simulink model "solarPV_grid_04_04"  (R2021a)
settings: Solver=FixedStepAuto  StartTime=0.0  StopTime=5  FixedStep=1e-6  RelTol=1e-3
libraries: spsIGBTDiodeLib x6, spsSeriesRLCBranchLib x6, slpidlib x4, spsCurrentMeasurementLib x4, spsVoltageMeasurementLib x2, simulink x2, spsGroundLib x1, spsPVArrayLib x1, spsdq0toabcLib x1, spsThreePhaseProgrammableVoltageSourceLib x1, spsThreePhaseVIMeasurementLib x1, spspowerguiLib x1
settings Model: Creator=user  LastModifiedBy=Arun Rahul S
settings SolverCC: AlgebraicLoopSolver=TrustRegion
settings DataIOCC: ReturnWorkspaceOutputs=off
settings DebuggingCC: SFMachineParentedDataDiag=warning  ArithmeticOperatorsInVariantConditions=warning
settings SFSimCC: SimUseLocalCustomCode=off  CustomCodeUndefinedFunction=UseInterfaceOnly
settings RTWCC: RTWUseLocalCustomCode=off

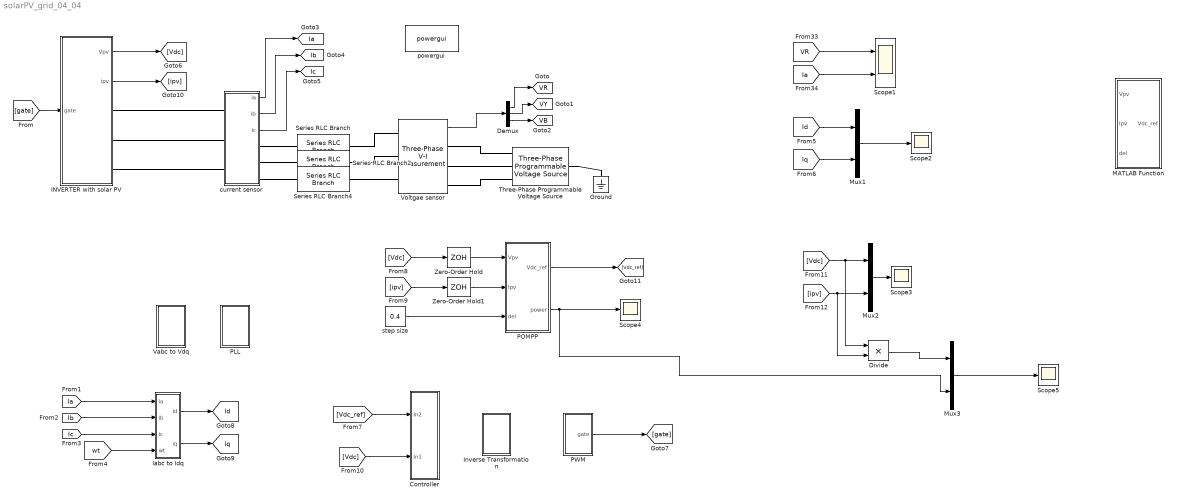
== system solarPV_grid_04_04 ==
  Controller : Subsystem
  Demux : Demux  Outputs=3
  Divide : Product  Inputs=**
  Ground : spsGroundLib/Ground  LConnTagsString=a
  INVERTER with solar PV : Subsystem
  Iabc to Idq : Subsystem
  Inverse Transformation : Subsystem
  MATLAB Function : MATLAB Function  TreatAsAtomicUnit=on
  Mux1 : Mux  Inputs=2
  Mux2 : Mux  Inputs=2
  Mux3 : Mux  Inputs=2
  PLL : Subsystem
  POMPP : MATLAB Function  TreatAsAtomicUnit=on
  PWM : Subsystem
  Scope1 : Scope  NumInputPorts=2
  Scope{2..5} (4 alike) : Scope
  Series RLC Branch : spsSeriesRLCBranchLib/Series RLC Branch  LConnTagsString=__new0  RConnTagsString=__new0  BranchType=RL  Resistance=0.6  Inductance=10e-3  SetiL0=off  InitialCurrent=0  Capacitance=1e-6  Setx0=off  InitialVoltage=0  Measurements=None
  Series RLC Branch2 : spsSeriesRLCBranchLib/Series RLC Branch  LConnTagsString=__new0  RConnTagsString=__new0  BranchType=RL  Resistance=0.6  Inductance=10e-3  SetiL0=off  InitialCurrent=0  Capacitance=1e-6  Setx0=off  InitialVoltage=0  Measurements=None
  Series RLC Branch4 : spsSeriesRLCBranchLib/Series RLC Branch  LConnTagsString=__new0  RConnTagsString=__new0  BranchType=RL  Resistance=0.6  Inductance=10e-3  SetiL0=off  InitialCurrent=0  Capacitance=1e-6  Setx0=off  InitialVoltage=0  Measurements=None
  Three-Phase Programmable Voltage Source : spsThreePhaseProgrammableVoltageSourceLib/Three-Phase Programmable Voltage Source  PositiveSequence="[400  0 50]"  VariationEntity=None  VariationType=Table of time-amplitude pairs  VariationTypeAlt=Step  VariationStep=0.5  VariationRate=10  VariationMagnitude=0.3  VariationFrequency=2  VariationTiming=[1 2]  VariationPhaseA=off  Amplitudes=[1 0.8 1.2 1.0]  TimeValues=[0 0.1 0.15 0.2]  HarmonicGeneration=off  HarmonicA=[3 0.2 -25 0]  HarmonicB=[2 0.15 35 2]  Timing="[0.05  3]"  BusType=swing  Pref=0  Qref=0  Qmin=-inf  Qmax=inf
  Vabc to Vdq : Subsystem
  Voltgae sensor : spsThreePhaseVIMeasurementLib/Three-Phase V-I Measurement  VoltageMeasurement=phase-to-ground  SetLabelV=off  LabelV=Vabc  Vpu=off  VpuLL=off  CurrentMeasurement=no  SetLabelI=off  LabelI=Iabc  Ipu=off  Pbase=100e6  Vbase=500e3  OutputType=Complex  PhasorSimulation=off  PSBequivalent=0
  Zero-Order Hold : ZeroOrderHold  SampleTime=10000e-6
  Zero-Order Hold1 : ZeroOrderHold  SampleTime=10000e-6
  current sensor : Subsystem
  powergui : spspowerguiLib/powergui  Priority=1  SimulationMode=Discrete  SampleTime=1e-6  frequency=60  Iterations=50  frequencyindice=50  Pbase=100e6  ErrMax=1e-4  UnitsV=kV  UnitsW=MW  buscounter=0  FunctionMessages=off  echomessages=off  EnableUseOfTLC=off  CurrentSourceSwitches=off  DisableSnubberDevices=off  DisableRonSwitches=off  DisableVfSwitches=off  DisplayEquations=off  AutomaticDiscreteSolvers=off  SolverType=Tustin/Backward Euler (TBE)  Interpol=off  ExternalGateDelay=off  methode=off  Ts=100  x0status=blocks  SPID=on  SwTol=0  HookPort=off  NonlinearTolerance=1e-4  nMaxIteration=100  ContinueOnMaxIteration=off  RestoreLinks=warning  ResistiveCurrentMeasurement=off  Frange=[0:2:500]  Ylog=off  Xlog=on  ShowGrid=off  save=off  variable=ZData  structure=ScopeData1  ZoomFFT=off  StartTime=0.91  cycles=4  DisplayStyle=1  fundamental=50  FreqAxis=off  MaxFrequency=1000  frequencyindicesteady=1  RmsSteady=1  display=off
  step size : Constant  Value=0.4
  tag scope: Ia=global, Ib=global, Ic=global, Id=global, Iq=global, VB=global, VR=global, VY=global
  wires:
  Demux/1 -> [VR]
  Demux/2 -> [VY]
  Demux/3 -> [VB]
  [VR] -> Scope1/1
  [Ia] -> Scope1/2
  current sensor/1(ia) -> [Ia]
  current sensor/2(ib) -> [Ib]
  current sensor/3(ic) -> [Ic]
  PWM/1(gate) -> [gate]
  [gate] -> INVERTER with solar PV/1(gate)
  [Iq] -> Mux1/2
  Mux1/1 -> Scope2/1
  [Id] -> Mux1/1
  [Ia] -> Iabc to Idq/1(ia)
  [Ib] -> Iabc to Idq/2(ib)
  [Ic] -> Iabc to Idq/3(ic)
  [wt] -> Iabc to Idq/4(wt)
  Iabc to Idq/1(id) -> [Id]
  Iabc to Idq/2(iq) -> [Iq]
  Voltgae sensor/1 -> Demux/1
  INVERTER with solar PV/1(Vpv) -> [Vdc]
  INVERTER with solar PV/2(ipv) -> [ipv]
  step size/1 -> POMPP/3(del)
  [Vdc] -> Zero-Order Hold/1
  [ipv] -> Zero-Order Hold1/1
  POMPP/1(Vdc_ref) -> [Vdc_ref]
  Zero-Order Hold/1 -> POMPP/1(Vpv)
  Zero-Order Hold1/1 -> POMPP/2(Ipv)
  [Vdc_ref] -> Controller/1(In2)
  [Vdc] -> Controller/2(In1)
  [Vdc] -> Divide/1, Mux2/1
  [ipv] -> Divide/2, Mux2/2
  Mux2/1 -> Scope3/1
  POMPP/2(power) -> Mux3/2, Scope4/1
  Divide/1 -> Mux3/1
  Mux3/1 -> Scope5/1
  connections:
  current sensor/LConn2 -- INVERTER with solar PV/RConn2
  current sensor/RConn2 -- Series RLC Branch2/LConn1
  current sensor/LConn3 -- INVERTER with solar PV/RConn3
  Series RLC Branch/LConn1 -- current sensor/RConn1
  Series RLC Branch4/LConn1 -- current sensor/RConn3
  Three-Phase Programmable Voltage Source/LConn1 -- Ground/LConn1
  Voltgae sensor/RConn1 -- Three-Phase Programmable Voltage Source/RConn1
  Voltgae sensor/RConn2 -- Three-Phase Programmable Voltage Source/RConn2
  Voltgae sensor/RConn3 -- Three-Phase Programmable Voltage Source/RConn3
  Series RLC Branch/RConn1 -- Voltgae sensor/LConn1
  Series RLC Branch2/RConn1 -- Voltgae sensor/LConn2
  Series RLC Branch4/RConn1 -- Voltgae sensor/LConn3
  INVERTER with solar PV/RConn1 -- current sensor/LConn1

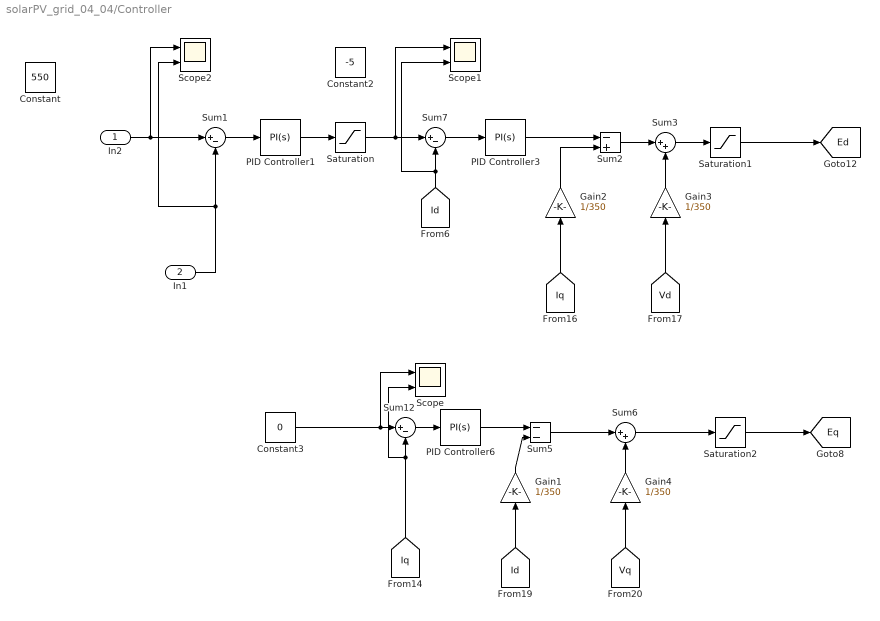
== system solarPV_grid_04_04/Controller ==
  In2 : Inport
  In1 : Inport  Port=2
  Constant : Constant  Value=550
  Constant2 : Constant  Value=-5
  Constant3 : Constant  Value=0
  Gain{1..4} (4 alike) : Gain  Gain=1/350
  PID Controller1 : slpidlib/PID Controller  Controller=PI  Form=Parallel  TimeDomain=Continuous-time  UseExternalTs=off  SampleTime=-1  IntegratorMethod=Forward Euler  FilterMethod=Forward Euler  ControllerParametersSource=internal  P=0.1  I=1  D=0  UseFilter=on  N=100  TunerSelectOption=Transfer Function Based (PID Tuner App)  InitialConditionSource=internal  InitialConditionForIntegrator=0  InitialConditionForFilter=0  DifferentiatorICPrevScaledInput=0  ExternalReset=none  TrackingMode=off  Kt=1  LimitOutput=off  SatLimitsSource=internal  UpperSaturationLimit=inf  LowerSaturationLimit=-inf  LinearizeAsGain=on  AntiWindupMode=none  Kb=1  POutMin=[]  POutMax=[]  IOutMin=[]  IOutMax=[]  DOutMin=[]  DOutMax=[]  NOutMin=[]  NOutMax=[]  SumOutMin=[]  SumOutMax=[]  SaturationOutMin=[]  SaturationOutMax=[]  PParamMin=[]  PParamMax=[]  IParamMin=[]  IParamMax=[]  DParamMin=[]  DParamMax=[]  NParamMin=[]  NParamMax=[]  KbParamMin=[]  KbParamMax=[]  KtParamMin=[]  KtParamMax=[]  KbOutMin=[]  KbOutMax=[]  KtOutMin=[]  KtOutMax=[]  IntegratorOutMin=[]  IntegratorOutMax=[]  FilterOutMin=[]  FilterOutMax=[]  SumI1OutMin=[]  SumI1OutMax=[]  SumI2OutMin=[]  SumI2OutMax=[]  SumI3OutMin=[]  SumI3OutMax=[]  SumI4OutMin=[]  SumI4OutMax=[]  SumDOutMin=[]  SumDOutMax=[]  DifferentiatorOutMin=[]  DifferentiatorOutMax=[]  FilterDiffOutCoefMin=[]  FilterDiffOutCoefMax=[]  ReciprocalOutMin=[]  ReciprocalOutMax=[]  SumDenOutMin=[]  SumDenOutMax=[]  SumNumOutMin=[]  SumNumOutMax=[]  DivideOutMin=[]  DivideOutMax=[]  UdiffTsProdOutMin=[]  UdiffTsProdOutMax=[]  NTsProdOutMin=[]  NTsProdOutMax=[]  UintegralTsProdOutMin=[]  UintegralTsProdOutMax=[]  UngainTsProdOutMin=[]  UngainTsProdOutMax=[]  IntegratorContinuousStateAttributes=''  IntegratorStateMustResolveToSignalObject=off  IntegratorRTWStateStorageClass=Auto  FilterContinuousStateAttributes=''  FilterStateMustResolveToSignalObject=off  FilterRTWStateStorageClass=Auto  ParallelPVariant=InternalParameters  IdealPVariant=Disabled  IVariant=InternalParameters  DVariant=Disabled  IntegratorVariant=Continuous  SatVariant=Disabled  AWVariant=Passthrough  PCopyVariant=Disabled  TRVariant=Disabled  FdbkBlocksVariant=Forward  IdealPFdbkVariant=Disabled  SatFdbkVariant=Disabled  DerivativeFilterVariant=Disabled  NVariant=Disabled  NCopyVariant=Disabled_SignalSpec  FilterICVariant=Disabled  IntegratorICVariant=InternalICs  ExternalResetVariant=Disabled  TRSumVariant=Passthrough  SumFdbkVariant=Disabled  SumVariant=Sum_PI  TsampFilterVariant=InternalTs  TsampNgainVariant=Passthrough  TsampIntegralVariant=Passthrough  ExternalSaturationOutDataTypeStr=Inherit: Same as second input
  PID Controller3 : slpidlib/PID Controller  Controller=PI  Form=Parallel  TimeDomain=Continuous-time  UseExternalTs=off  SampleTime=-1  IntegratorMethod=Forward Euler  FilterMethod=Forward Euler  ControllerParametersSource=internal  P=1  I=1  D=0  UseFilter=on  N=100  TunerSelectOption=Transfer Function Based (PID Tuner App)  InitialConditionSource=internal  InitialConditionForIntegrator=0  InitialConditionForFilter=0  DifferentiatorICPrevScaledInput=0  ExternalReset=none  TrackingMode=off  Kt=1  LimitOutput=off  SatLimitsSource=internal  UpperSaturationLimit=inf  LowerSaturationLimit=-inf  LinearizeAsGain=on  AntiWindupMode=none  Kb=1  POutMin=[]  POutMax=[]  IOutMin=[]  IOutMax=[]  DOutMin=[]  DOutMax=[]  NOutMin=[]  NOutMax=[]  SumOutMin=[]  SumOutMax=[]  SaturationOutMin=[]  SaturationOutMax=[]  PParamMin=[]  PParamMax=[]  IParamMin=[]  IParamMax=[]  DParamMin=[]  DParamMax=[]  NParamMin=[]  NParamMax=[]  KbParamMin=[]  KbParamMax=[]  KtParamMin=[]  KtParamMax=[]  KbOutMin=[]  KbOutMax=[]  KtOutMin=[]  KtOutMax=[]  IntegratorOutMin=[]  IntegratorOutMax=[]  FilterOutMin=[]  FilterOutMax=[]  SumI1OutMin=[]  SumI1OutMax=[]  SumI2OutMin=[]  SumI2OutMax=[]  SumI3OutMin=[]  SumI3OutMax=[]  SumI4OutMin=[]  SumI4OutMax=[]  SumDOutMin=[]  SumDOutMax=[]  DifferentiatorOutMin=[]  DifferentiatorOutMax=[]  FilterDiffOutCoefMin=[]  FilterDiffOutCoefMax=[]  ReciprocalOutMin=[]  ReciprocalOutMax=[]  SumDenOutMin=[]  SumDenOutMax=[]  SumNumOutMin=[]  SumNumOutMax=[]  DivideOutMin=[]  DivideOutMax=[]  UdiffTsProdOutMin=[]  UdiffTsProdOutMax=[]  NTsProdOutMin=[]  NTsProdOutMax=[]  UintegralTsProdOutMin=[]  UintegralTsProdOutMax=[]  UngainTsProdOutMin=[]  UngainTsProdOutMax=[]  IntegratorContinuousStateAttributes=''  IntegratorStateMustResolveToSignalObject=off  IntegratorRTWStateStorageClass=Auto  FilterContinuousStateAttributes=''  FilterStateMustResolveToSignalObject=off  FilterRTWStateStorageClass=Auto  ParallelPVariant=InternalParameters  IdealPVariant=Disabled  IVariant=InternalParameters  DVariant=Disabled  IntegratorVariant=Continuous  SatVariant=Disabled  AWVariant=Passthrough  PCopyVariant=Disabled  TRVariant=Disabled  FdbkBlocksVariant=Forward  IdealPFdbkVariant=Disabled  SatFdbkVariant=Disabled  DerivativeFilterVariant=Disabled  NVariant=Disabled  NCopyVariant=Disabled_SignalSpec  FilterICVariant=Disabled  IntegratorICVariant=InternalICs  ExternalResetVariant=Disabled  TRSumVariant=Passthrough  SumFdbkVariant=Disabled  SumVariant=Sum_PI  TsampFilterVariant=InternalTs  TsampNgainVariant=Passthrough  TsampIntegralVariant=Passthrough  ExternalSaturationOutDataTypeStr=Inherit: Same as second input
  PID Controller6 : slpidlib/PID Controller  Controller=PI  Form=Parallel  TimeDomain=Continuous-time  UseExternalTs=off  SampleTime=-1  IntegratorMethod=Forward Euler  FilterMethod=Forward Euler  ControllerParametersSource=internal  P=1  I=1  D=0  UseFilter=on  N=100  TunerSelectOption=Transfer Function Based (PID Tuner App)  InitialConditionSource=internal  InitialConditionForIntegrator=0  InitialConditionForFilter=0  DifferentiatorICPrevScaledInput=0  ExternalReset=none  TrackingMode=off  Kt=1  LimitOutput=off  SatLimitsSource=internal  UpperSaturationLimit=inf  LowerSaturationLimit=-inf  LinearizeAsGain=on  AntiWindupMode=none  Kb=1  POutMin=[]  POutMax=[]  IOutMin=[]  IOutMax=[]  DOutMin=[]  DOutMax=[]  NOutMin=[]  NOutMax=[]  SumOutMin=[]  SumOutMax=[]  SaturationOutMin=[]  SaturationOutMax=[]  PParamMin=[]  PParamMax=[]  IParamMin=[]  IParamMax=[]  DParamMin=[]  DParamMax=[]  NParamMin=[]  NParamMax=[]  KbParamMin=[]  KbParamMax=[]  KtParamMin=[]  KtParamMax=[]  KbOutMin=[]  KbOutMax=[]  KtOutMin=[]  KtOutMax=[]  IntegratorOutMin=[]  IntegratorOutMax=[]  FilterOutMin=[]  FilterOutMax=[]  SumI1OutMin=[]  SumI1OutMax=[]  SumI2OutMin=[]  SumI2OutMax=[]  SumI3OutMin=[]  SumI3OutMax=[]  SumI4OutMin=[]  SumI4OutMax=[]  SumDOutMin=[]  SumDOutMax=[]  DifferentiatorOutMin=[]  DifferentiatorOutMax=[]  FilterDiffOutCoefMin=[]  FilterDiffOutCoefMax=[]  ReciprocalOutMin=[]  ReciprocalOutMax=[]  SumDenOutMin=[]  SumDenOutMax=[]  SumNumOutMin=[]  SumNumOutMax=[]  DivideOutMin=[]  DivideOutMax=[]  UdiffTsProdOutMin=[]  UdiffTsProdOutMax=[]  NTsProdOutMin=[]  NTsProdOutMax=[]  UintegralTsProdOutMin=[]  UintegralTsProdOutMax=[]  UngainTsProdOutMin=[]  UngainTsProdOutMax=[]  IntegratorContinuousStateAttributes=''  IntegratorStateMustResolveToSignalObject=off  IntegratorRTWStateStorageClass=Auto  FilterContinuousStateAttributes=''  FilterStateMustResolveToSignalObject=off  FilterRTWStateStorageClass=Auto  ParallelPVariant=InternalParameters  IdealPVariant=Disabled  IVariant=InternalParameters  DVariant=Disabled  IntegratorVariant=Continuous  SatVariant=Disabled  AWVariant=Passthrough  PCopyVariant=Disabled  TRVariant=Disabled  FdbkBlocksVariant=Forward  IdealPFdbkVariant=Disabled  SatFdbkVariant=Disabled  DerivativeFilterVariant=Disabled  NVariant=Disabled  NCopyVariant=Disabled_SignalSpec  FilterICVariant=Disabled  IntegratorICVariant=InternalICs  ExternalResetVariant=Disabled  TRSumVariant=Passthrough  SumFdbkVariant=Disabled  SumVariant=Sum_PI  TsampFilterVariant=InternalTs  TsampNgainVariant=Passthrough  TsampIntegralVariant=Passthrough  ExternalSaturationOutDataTypeStr=Inherit: Same as second input
  Saturation : Saturate  UpperLimit=10  LowerLimit=-10
  Saturation1 : Saturate  UpperLimit=1.2  LowerLimit=-1.2
  Saturation2 : Saturate  UpperLimit=1.2  LowerLimit=-1.2
  Scope : Scope  NumInputPorts=2
  Scope1 : Scope  NumInputPorts=2
  Scope2 : Scope  NumInputPorts=2
  Sum1 : Sum  Inputs=|+-
  Sum12 : Sum  Inputs=|+-
  Sum2 : Sum  Inputs=-+
  Sum3 : Sum  Inputs=|++
  Sum5 : Sum  Inputs=--
  Sum6 : Sum  Inputs=|++
  Sum7 : Sum  Inputs=|+-
  tag scope: Ed=global, Eq=global
  wires:
  [Id] -> Scope1/2, Sum7/2
  [Id] -> Gain1/1
  In1/1 -> Scope2/2, Sum1/2
  Sum2/1 -> Sum3/1
  Sum1/1 -> PID Controller1/1
  [Iq] -> Scope/2, Sum12/2
  Sum12/1 -> PID Controller6/1
  Constant3/1 -> Scope/1, Sum12/1
  Sum7/1 -> PID Controller3/1
  Sum6/1 -> Saturation2/1
  Sum5/1 -> Sum6/1
  Sum3/1 -> Saturation1/1
  PID Controller3/1 -> Sum2/1
  PID Controller6/1 -> Sum5/1
  [Iq] -> Gain2/1
  Saturation1/1 -> [Ed]
  Saturation2/1 -> [Eq]
  [Vd] -> Gain3/1
  Gain3/1 -> Sum3/2
  [Vq] -> Gain4/1
  Gain4/1 -> Sum6/2
  Gain2/1 -> Sum2/2
  Gain1/1 -> Sum5/2
  PID Controller1/1 -> Saturation/1
  Saturation/1 -> Scope1/1, Sum7/1
  In2/1 -> Scope2/1, Sum1/1

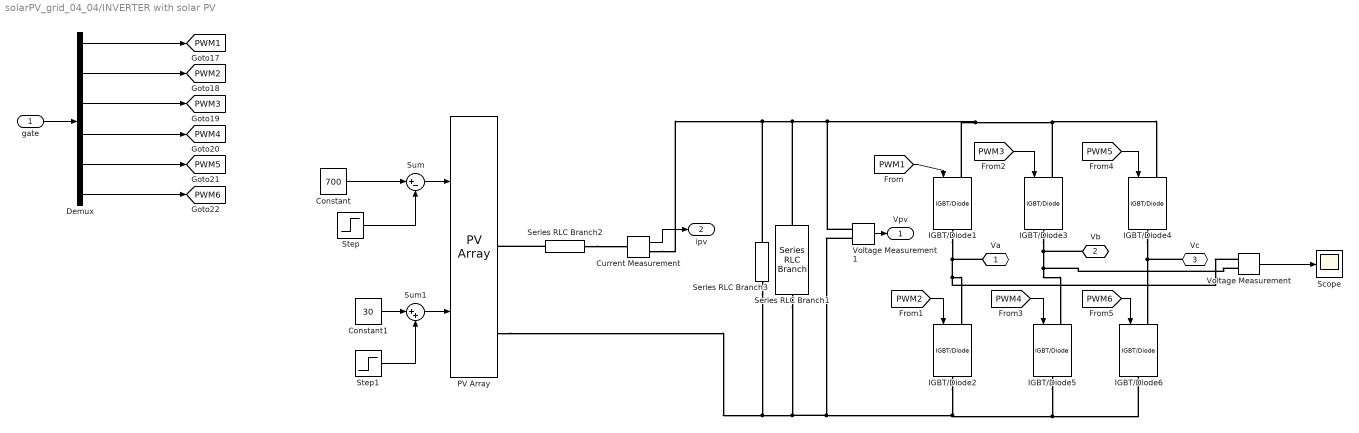
== system solarPV_grid_04_04/INVERTER with solar PV ==
  gate : Inport
  Constant : Constant  Value=700
  Constant1 : Constant  Value=30
  Current Measurement : spsCurrentMeasurementLib/Current Measurement  PhasorSimulation=off  OutputType=Complex  PSBequivalent=0
  Demux : Demux  Outputs=6
  IGBT/Diode{1..6} (6 alike) : spsIGBTDiodeLib/IGBT//Diode  Ron=1e-3  Rs=1e5  Cs=inf  Measurements=off
  PV Array : spsPVArrayLib/PV Array  Npar=1  Nser=24  PlotType=array @ 1000 W/m2 & specified temperatures  S_vec="[ 1000  500  100 ]"  Temp_C_vec="[ 45 25  ]"  ModuleName=User-defined  PlotWhenSelected=off  Pm=213.15  Ncell=60  Voc=36.3  Isc=7.84  Vm=29  Im=7.35  beta_Voc_pc=-0.36099  alpha_Isc_pc=0.102  beta_Voc=-0.13104  alpha_Isc=0.0079968  IL=7.8654  I0=2.9273e-10  nI=0.98119  Rsh=313.0553  Rs=0.39381  RobustModel=off  RobustCellTemperature=313.3991  BAL=on  Tc=1e-6  Tfilter=5e-5
  Scope : Scope
  Series RLC Branch1 : spsSeriesRLCBranchLib/Series RLC Branch  LConnTagsString=__new0  RConnTagsString=__new0  BranchType=RC  Resistance=0.1  Inductance=1e-3  SetiL0=off  InitialCurrent=0  Capacitance=2200e-6  Setx0=on  InitialVoltage=24*36.3  Measurements=Branch voltage
  Series RLC Branch2 : spsSeriesRLCBranchLib/Series RLC Branch  LConnTagsString=__new0  RConnTagsString=__new0  BranchType=R  Resistance=0.5  Inductance=1e-3  SetiL0=off  InitialCurrent=0  Capacitance=4400e-6  Setx0=off  InitialVoltage=0  Measurements=Branch voltage
  Series RLC Branch3 : spsSeriesRLCBranchLib/Series RLC Branch  LConnTagsString=__new0  RConnTagsString=__new0  BranchType=R  Resistance=1000  Inductance=1e-3  SetiL0=off  InitialCurrent=0  Capacitance=4400e-6  Setx0=off  InitialVoltage=0  Measurements=Branch voltage
  Step : Step  Time=3  After=200  SampleTime=0
  Step1 : Step  Time=4  After=10  SampleTime=0
  Sum : Sum  Inputs=|+-
  Sum1 : Sum  Inputs=|++
  Voltage Measurement : spsVoltageMeasurementLib/Voltage Measurement  PhasorSimulation=off  OutputType=Complex  PSBequivalent=0
  Voltage Measurement1 : spsVoltageMeasurementLib/Voltage Measurement  PhasorSimulation=off  OutputType=Complex  PSBequivalent=0
  Va : PMIOPort  Side=Right
  Vb : PMIOPort  Port=2  Side=Right
  Vc : PMIOPort  Port=3  Side=Right
  Vpv : Outport
  ipv : Outport  Port=2
  tag scope: PWM1=global, PWM2=global, PWM3=global, PWM4=global, PWM5=global, PWM6=global
  wires:
  [PWM2] -> IGBT/Diode2/1
  [PWM6] -> IGBT/Diode6/1
  [PWM4] -> IGBT/Diode5/1
  [PWM5] -> IGBT/Diode4/1
  [PWM3] -> IGBT/Diode3/1
  Voltage Measurement/1 -> Scope/1
  gate/1 -> Demux/1
  [PWM1] -> IGBT/Diode1/1
  Demux/1 -> [PWM1]
  Demux/2 -> [PWM2]
  Demux/3 -> [PWM3]
  Demux/4 -> [PWM4]
  Demux/5 -> [PWM5]
  Demux/6 -> [PWM6]
  Current Measurement/1 -> ipv/1
  Sum/1 -> PV Array/1
  Constant/1 -> Sum/1
  Step/1 -> Sum/2
  Constant1/1 -> Sum1/1
  Step1/1 -> Sum1/2
  Sum1/1 -> PV Array/2
  Voltage Measurement1/1 -> Vpv/1
  connections:
  IGBT/Diode3/RConn1 -- Vb/RConn1 -- Voltage Measurement/LConn2 -- IGBT/Diode5/LConn1
  IGBT/Diode2/RConn1 -- Voltage Measurement1/LConn2 -- PV Array/RConn2 -- Series RLC Branch3/RConn1 -- Series RLC Branch1/RConn1 -- IGBT/Diode5/RConn1 -- IGBT/Diode6/RConn1
  IGBT/Diode4/RConn1 -- Vc/RConn1 -- IGBT/Diode6/LConn1
  IGBT/Diode1/RConn1 -- Voltage Measurement/LConn1 -- IGBT/Diode2/LConn1 -- Va/RConn1
  IGBT/Diode3/LConn1 -- Series RLC Branch1/LConn1 -- Series RLC Branch3/LConn1 -- Current Measurement/RConn1 -- Voltage Measurement1/LConn1 -- IGBT/Diode1/LConn1 -- IGBT/Diode4/LConn1
  Series RLC Branch2/RConn1 -- PV Array/RConn1
  Series RLC Branch2/LConn1 -- Current Measurement/LConn1

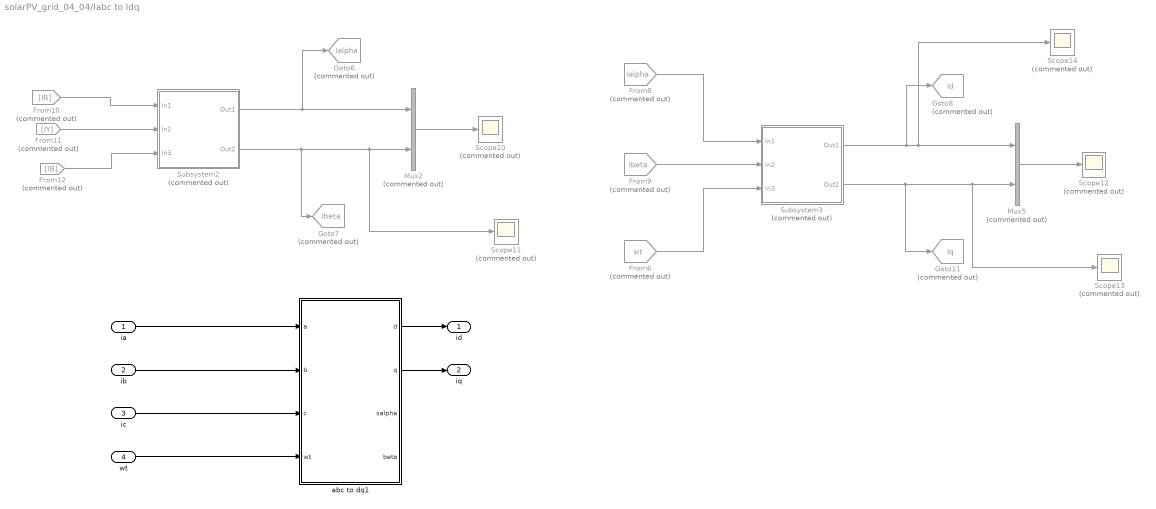
== system solarPV_grid_04_04/Iabc to Idq ==
  ia : Inport
  ib : Inport  Port=2
  ic : Inport  Port=3
  wt : Inport  Port=4
  From10 : From  Commented=on  GotoTag=IR  TagVisibility=global
  From11 : From  Commented=on  GotoTag=IY  TagVisibility=global
  From12 : From  Commented=on  GotoTag=IB  TagVisibility=global
  From6 : From  Commented=on  GotoTag=wt  TagVisibility=global
  From8 : From  Commented=on  GotoTag=Ialpha  TagVisibility=global
  From9 : From  Commented=on  GotoTag=Ibeta  TagVisibility=global
  Goto11 : Goto  Commented=on  GotoTag=Iq  TagVisibility=global
  Goto6 : Goto  Commented=on  GotoTag=Ialpha  TagVisibility=global
  Goto7 : Goto  Commented=on  GotoTag=Ibeta  TagVisibility=global
  Goto8 : Goto  Commented=on  GotoTag=Id  TagVisibility=global
  Mux2 : Mux  Commented=on  Inputs=2
  Mux5 : Mux  Commented=on  Inputs=2
  Scope{10..14} (5 alike) : Scope  Commented=on
  Subsystem2 : Subsystem  Commented=on
  Subsystem3 : Subsystem  Commented=on
  abc to dq1 : Subsystem
  id : Outport
  iq : Outport  Port=2
  wires:
  Subsystem2/2(Out2) -> Goto7/1, Scope11/1, Mux2/2
  From8/1 -> Subsystem3/1(In1)
  From10/1 -> Subsystem2/1(In1)
  Mux5/1 -> Scope12/1
  Subsystem2/1(Out1) -> Goto6/1, Mux2/1
  From11/1 -> Subsystem2/2(In2)
  Subsystem3/1(Out1) -> Goto8/1, Scope14/1, Mux5/1
  From6/1 -> Subsystem3/3(In3)
  Subsystem3/2(Out2) -> Goto11/1, Scope13/1, Mux5/2
  From9/1 -> Subsystem3/2(In2)
  Mux2/1 -> Scope10/1
  From12/1 -> Subsystem2/3(In3)
  ia/1 -> abc to dq1/1(a)
  ib/1 -> abc to dq1/2(b)
  ic/1 -> abc to dq1/3(c)
  wt/1 -> abc to dq1/4(wt)
  abc to dq1/2(q) -> iq/1
  abc to dq1/1(d) -> id/1

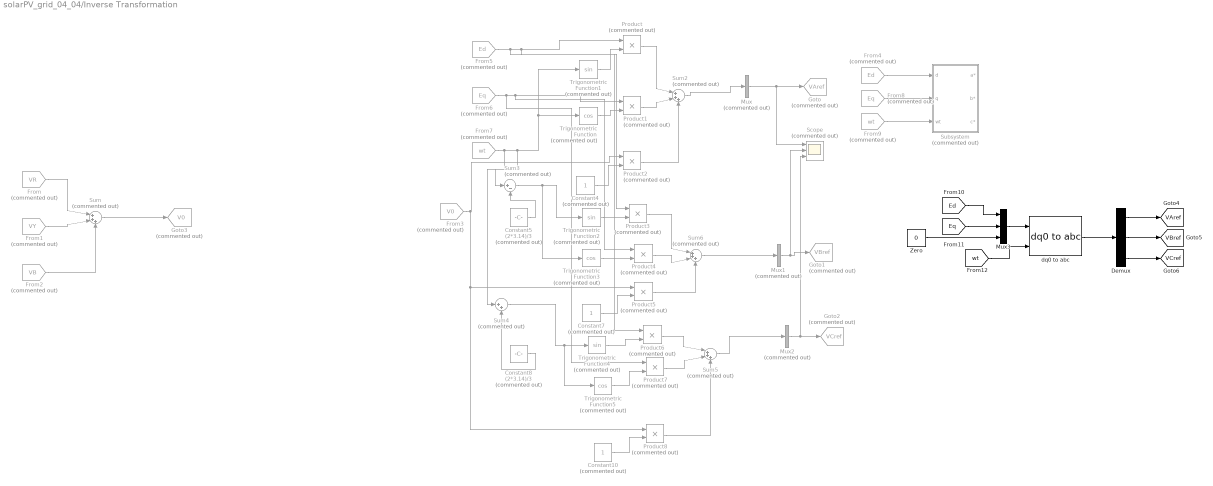
== system solarPV_grid_04_04/Inverse Transformation ==
  Constant10 : Constant  Commented=on
  Constant4 : Constant  Commented=on
  Constant5 : Constant  Commented=on  Value=(2*3.14)/3
  Constant7 : Constant  Commented=on
  Constant8 : Constant  Commented=on  Value=(2*3.14)/3
  Demux : Demux  Outputs=3
  From : From  Commented=on  GotoTag=VR  TagVisibility=global
  From1 : From  Commented=on  GotoTag=VY  TagVisibility=global
  From2 : From  Commented=on  GotoTag=VB  TagVisibility=global
  From3 : From  Commented=on  GotoTag=V0  TagVisibility=global
  From4 : From  Commented=on  GotoTag=Ed  TagVisibility=global
  From5 : From  Commented=on  GotoTag=Ed  TagVisibility=global
  From6 : From  Commented=on  GotoTag=Eq  TagVisibility=global
  From7 : From  Commented=on  GotoTag=wt  TagVisibility=global
  From8 : From  Commented=on  GotoTag=Eq  TagVisibility=global
  From9 : From  Commented=on  GotoTag=wt  TagVisibility=global
  Goto : Goto  Commented=on  GotoTag=VAref  TagVisibility=global
  Goto1 : Goto  Commented=on  GotoTag=VBref  TagVisibility=global
  Goto2 : Goto  Commented=on  GotoTag=VCref  TagVisibility=global
  Goto3 : Goto  Commented=on  GotoTag=V0  TagVisibility=global
  Mux : Mux  Commented=on  Inputs=1
  Mux1 : Mux  Commented=on  Inputs=1
  Mux2 : Mux  Commented=on  Inputs=1
  Mux3 : Mux  Inputs=3
  Product{,1..8} (9 alike) : Product  Commented=on
  Scope : Scope  Commented=on  NumInputPorts=3
  Subsystem : Subsystem  Commented=on
  Sum{,2,5..6} (4 alike) : Sum  Commented=on  Inputs=|+++
  Sum3 : Sum  Commented=on  Inputs=|+-
  Sum4 : Sum  Commented=on  Inputs=|++
  Trigonometric Function : Trigonometry  Commented=on  Operator=cos
  Trigonometric Function1 : Trigonometry  Commented=on
  Trigonometric Function2 : Trigonometry  Commented=on
  Trigonometric Function3 : Trigonometry  Commented=on  Operator=cos
  Trigonometric Function4 : Trigonometry  Commented=on
  Trigonometric Function5 : Trigonometry  Commented=on  Operator=cos
  Zero : Constant  Value=0
  dq0 to abc : spsdq0toabcLib/dq0 to abc  Alignment=Aligned with phase A axis
  tag scope: VAref=global, VBref=global, VCref=global
  wires:
  Constant5/1 -> Sum3/2
  Product5/1 -> Sum6/3
  Trigonometric Function/1 -> Product1/2
  From6/1 -> Product7/1, Product4/1, Product1/1
  From5/1 -> Product6/1, Product3/1, Product/1
  Constant10/1 -> Product8/2
  Constant4/1 -> Product2/2
  Product4/1 -> Sum6/2
  Sum3/1 -> Trigonometric Function3/1, Trigonometric Function2/1
  Trigonometric Function2/1 -> Product3/2
  Product3/1 -> Sum6/1
  Trigonometric Function1/1 -> Product/2
  From7/1 -> Sum3/1, Sum4/1, Trigonometric Function/1, Trigonometric Function1/1
  Trigonometric Function5/1 -> Product7/2
  Product1/1 -> Sum2/2
  Product6/1 -> Sum5/1
  Product2/1 -> Sum2/3
  Product/1 -> Sum2/1
  Trigonometric Function4/1 -> Product6/2
  Constant7/1 -> Product5/2
  Sum4/1 -> Trigonometric Function5/1, Trigonometric Function4/1
  Product7/1 -> Sum5/2
  Trigonometric Function3/1 -> Product4/2
  Constant8/1 -> Sum4/2
  Product8/1 -> Sum5/3
  Sum2/1 -> Mux/1
  Sum6/1 -> Mux1/1
  Sum5/1 -> Mux2/1
  Mux/1 -> Scope/1, Goto/1
  Mux1/1 -> Scope/2, Goto1/1
  Mux2/1 -> Scope/3, Goto2/1
  From/1 -> Sum/1
  From1/1 -> Sum/2
  From2/1 -> Sum/3
  Sum/1 -> Goto3/1
  From3/1 -> Product8/1, Product5/1, Product2/1
  From4/1 -> Subsystem/1(d)
  From8/1 -> Subsystem/2(q)
  From9/1 -> Subsystem/3(wt)
  Mux3/1 -> dq0 to abc/1
  Zero/1 -> Mux3/3
  [wt] -> dq0 to abc/2
  Demux/2 -> [VBref]
  Demux/1 -> [VAref]
  Demux/3 -> [VCref]
  dq0 to abc/1 -> Demux/1
  [Eq] -> Mux3/2
  [Ed] -> Mux3/1

== system solarPV_grid_04_04/PLL ==
  PLL : Subsystem
  tag scope: w=global, wt=global
  wires:
  [Vd] -> ?
  [Vq] -> PLL/1(vq)
  PLL/1(theta) -> [wt]
  PLL/2(w) -> [w]

== system solarPV_grid_04_04/PWM ==
  Mux : Mux  Inputs=6
  SVPWM : Subsystem  Commented=on
  Subsystem : Subsystem
  gate : Outport  VectorParamsAs1DForOutWhenUnconnected=off
  wires:
  [VCref] -> Subsystem/3(VCref)
  [VAref] -> Subsystem/1("VAref ")
  [VBref] -> Subsystem/2(VBref)
  Subsystem/1(PWM1) -> Mux/1
  Subsystem/2(PWM2) -> Mux/2
  Subsystem/3(PWM3) -> Mux/3
  Subsystem/4(PWM4) -> Mux/4
  Subsystem/5(PWM5) -> Mux/5
  Subsystem/6(PWM6) -> Mux/6
  Mux/1 -> gate/1

== system solarPV_grid_04_04/Vabc to Vdq ==
  From10 : From  Commented=on  GotoTag=wt  TagVisibility=global
  From8 : From  Commented=on  GotoTag=Valpha
  From9 : From  Commented=on  GotoTag=Vbeta
  Mux5 : Mux  Inputs=2
  Scope12 : Scope
  Subsystem3 : Subsystem  Commented=on
  abc to dq1 : Subsystem
  tag scope: Vd=global, Vq=global
  wires:
  From9/1 -> Subsystem3/2(In2)
  From8/1 -> Subsystem3/1(In1)
  From10/1 -> Subsystem3/3(In3)
  Mux5/1 -> Scope12/1
  [VR] -> abc to dq1/1(Vsa)
  [VY] -> abc to dq1/2(Vsb)
  [VB] -> abc to dq1/3(Vsc)
  [wt] -> abc to dq1/4(speed(w))
  [Vd] -> Mux5/1
  [Vq] -> Mux5/2
  abc to dq1/2(Vsq) -> [Vq]
  abc to dq1/1(Vsd) -> [Vd]

== system solarPV_grid_04_04/current sensor ==
  Current Measurement : spsCurrentMeasurementLib/Current Measurement  PhasorSimulation=off  OutputType=Complex  PSBequivalent=0
  Current Measurement1 : spsCurrentMeasurementLib/Current Measurement  PhasorSimulation=off  OutputType=Complex  PSBequivalent=0
  Current Measurement2 : spsCurrentMeasurementLib/Current Measurement  PhasorSimulation=off  OutputType=Complex  PSBequivalent=0
  a : PMIOPort  Side=Left
  a' : PMIOPort  Port=2  Side=Right
  b : PMIOPort  Port=3  Side=Left
  b' : PMIOPort  Port=4  Side=Right
  c : PMIOPort  Port=5  Side=Left
  c' : PMIOPort  Port=6  Side=Right
  ia : Outport
  ib : Outport  Port=2
  ic : Outport  Port=3
  wires:
  Current Measurement2/1 -> ic/1
  Current Measurement1/1 -> ib/1
  Current Measurement/1 -> ia/1
  connections:
  Current Measurement/RConn1 -- a/RConn1
  Current Measurement/LConn1 -- a'/RConn1
  b/RConn1 -- Current Measurement1/RConn1
  Current Measurement1/LConn1 -- b'/RConn1
  Current Measurement2/LConn1 -- c'/RConn1
  c/RConn1 -- Current Measurement2/RConn1

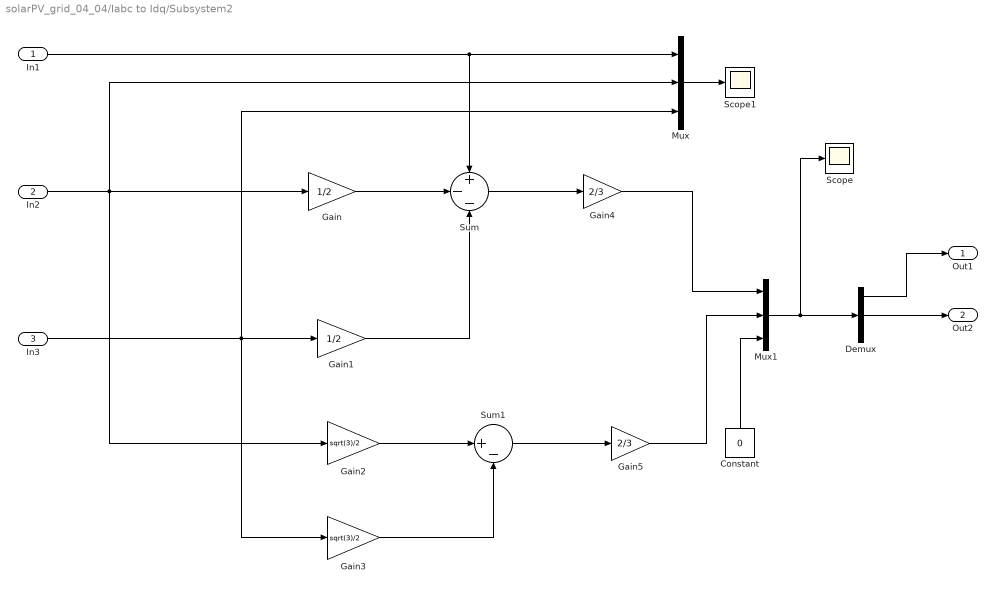
== system solarPV_grid_04_04/Iabc to Idq/Subsystem2 ==
  In1 : Inport
  In2 : Inport  Port=2
  In3 : Inport  Port=3
  Constant : Constant  Value=0
  Demux : Demux  Outputs=3
  Gain : Gain  Gain=1/2
  Gain1 : Gain  Gain=1/2
  Gain2 : Gain  Gain=sqrt(3)/2
  Gain3 : Gain  Gain=sqrt(3)/2
  Gain4 : Gain  Gain=2/3
  Gain5 : Gain  Gain=2/3
  Mux : Mux  Inputs=3
  Mux1 : Mux  Inputs=3
  Scope : Scope
  Scope1 : Scope
  Sum : Sum  Inputs=+--
  Sum1 : Sum  Inputs=|+-
  Out1 : Outport  VectorParamsAs1DForOutWhenUnconnected=off
  Out2 : Outport  Port=2  VectorParamsAs1DForOutWhenUnconnected=off
  wires:
  In1/1 -> Sum/1, Mux/1
  In2/1 -> Gain2/1, Mux/2, Gain/1
  In3/1 -> Mux/3, Gain3/1, Gain1/1
  Gain/1 -> Sum/2
  Sum/1 -> Gain4/1
  Sum1/1 -> Gain5/1
  Gain1/1 -> Sum/3
  Gain2/1 -> Sum1/1
  Gain3/1 -> Sum1/2
  Gain4/1 -> Mux1/1
  Gain5/1 -> Mux1/2
  Constant/1 -> Mux1/3
  Mux1/1 -> Scope/1, Demux/1
  Demux/1 -> Out1/1
  Demux/2 -> Out2/1
  Mux/1 -> Scope1/1

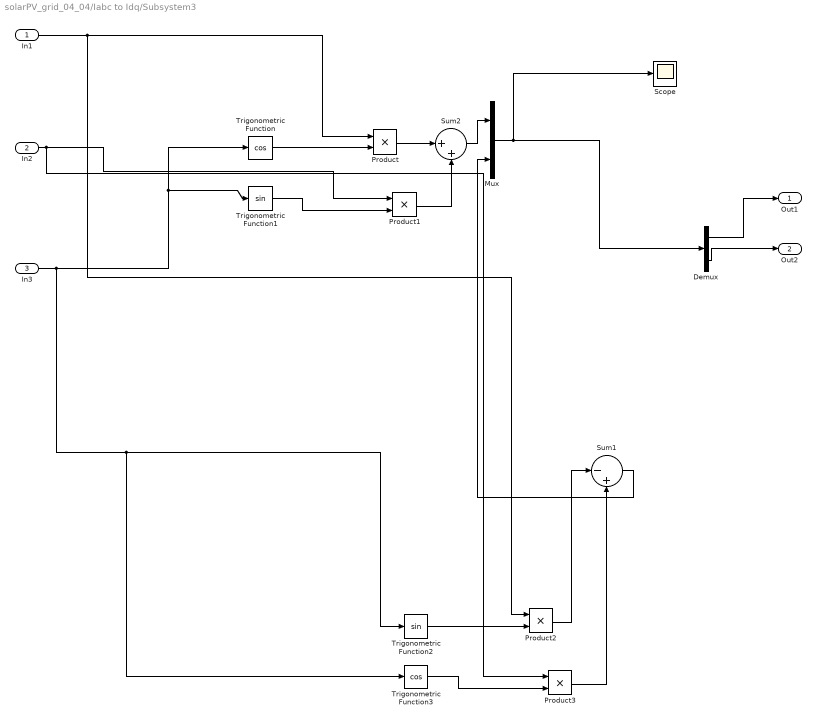
== system solarPV_grid_04_04/Iabc to Idq/Subsystem3 ==
  In1 : Inport
  In2 : Inport  Port=2
  In3 : Inport  Port=3
  Demux : Demux  Outputs=2
  Mux : Mux  Inputs=2
  Product{,1..3} (4 alike) : Product
  Scope : Scope
  Sum1 : Sum  Inputs=|-+
  Sum2 : Sum  Inputs=|++
  Trigonometric Function : Trigonometry  Operator=cos
  Trigonometric Function1 : Trigonometry
  Trigonometric Function2 : Trigonometry
  Trigonometric Function3 : Trigonometry  Operator=cos
  Out1 : Outport  VectorParamsAs1DForOutWhenUnconnected=off
  Out2 : Outport  Port=2  VectorParamsAs1DForOutWhenUnconnected=off
  wires:
  Demux/1 -> Out1/1
  Demux/2 -> Out2/1
  In3/1 -> Trigonometric Function3/1, Trigonometric Function2/1, Trigonometric Function1/1, Trigonometric Function/1
  Trigonometric Function/1 -> Product/2
  Product/1 -> Sum2/1
  In2/1 -> Product3/1, Product1/1
  Trigonometric Function1/1 -> Product1/2
  Product1/1 -> Sum2/2
  Product3/1 -> Sum1/2
  Product2/1 -> Sum1/1
  Trigonometric Function3/1 -> Product3/2
  Trigonometric Function2/1 -> Product2/2
  In1/1 -> Product2/1, Product/1
  Mux/1 -> Scope/1, Demux/1
  Sum2/1 -> Mux/1
  Sum1/1 -> Mux/2

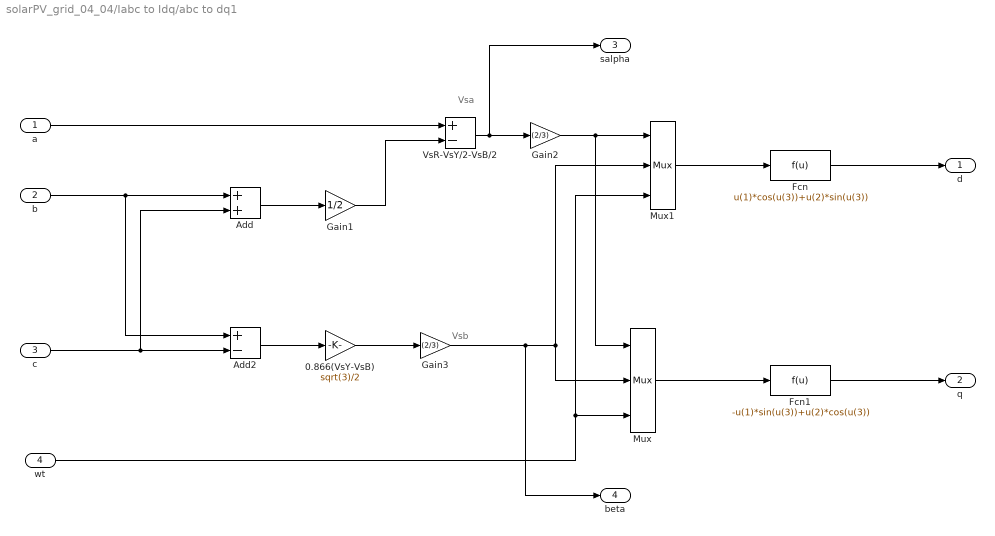
== system solarPV_grid_04_04/Iabc to Idq/abc to dq1 ==
  note: Vsa
  note: Vsb
  a : Inport
  b : Inport  Port=2
  c : Inport  Port=3
  wt : Inport  Port=4
  0.866(VsY-VsB) : Gain  Gain=sqrt(3)/2
  Add : Sum
  Add2 : Sum  Inputs=+-
  Fcn : Fcn  Expr=u(1)*cos(u(3))+u(2)*sin(u(3))
  Fcn1 : Fcn  Expr=-u(1)*sin(u(3))+u(2)*cos(u(3))
  Gain1 : Gain  Gain=1/2
  Gain2 : Gain  Gain=(2/3)
  Gain3 : Gain  Gain=(2/3)
  Mux : Mux  Inputs=3
  Mux1 : Mux  Inputs=3
  VsR-VsY/2-VsB/2 : Sum  Inputs=+-
  d : Outport
  q : Outport  Port=2
  salpha : Outport  Port=3
  beta : Outport  Port=4
  wires:
  wt/1 -> Mux/3, Mux1/3
  VsR-VsY/2-VsB/2/1 -> Gain2/1, salpha/1
  0.866(VsY-VsB)/1 -> Gain3/1
  Fcn1/1 -> q/1
  Fcn/1 -> d/1
  b/1 -> Add/1, Add2/1
  a/1 -> VsR-VsY/2-VsB/2/1
  c/1 -> Add2/2, Add/2
  Add2/1 -> 0.866(VsY-VsB)/1
  Add/1 -> Gain1/1
  Gain1/1 -> VsR-VsY/2-VsB/2/2
  Mux/1 -> Fcn1/1
  Mux1/1 -> Fcn/1
  Gain2/1 -> Mux1/1, Mux/1
  Gain3/1 -> Mux/2, Mux1/2, beta/1

== system solarPV_grid_04_04/Inverse Transformation/Subsystem ==
  d : Inport
  q : Inport  Port=2
  wt : Inport  Port=3
  Fcn : Fcn  Expr=u(1)*cos(u(3))-u(2)*sin(u(3))
  Fcn1 : Fcn  Expr=u(1)*sin(u(3))+u(2)*cos(u(3))
  Fcn2 : Fcn  Expr=u(1)*(2/3)
  Fcn3 : Fcn  Expr=-u(1)*(1/3)+(1/sqrt(3))*u(2)
  Fcn4 : Fcn  Expr=-u(1)*(1/3)-(1/sqrt(3))*u(2)
  Mux : Mux  Inputs=3
  Mux1 : Mux  Inputs=3
  Mux2 : Mux  Inputs=2
  Mux3 : Mux  Inputs=2
  a* : Outport
  b* : Outport  Port=2
  c* : Outport  Port=3
  wires:
  Mux/1 -> Fcn/1
  q/1 -> Mux/2, Mux1/2
  Mux1/1 -> Fcn1/1
  d/1 -> Mux/1, Mux1/1
  wt/1 -> Mux1/3, Mux/3
  Fcn/1 -> Mux2/1, Mux3/1, Fcn2/1
  Mux2/1 -> Fcn3/1
  Fcn1/1 -> Mux3/2, Mux2/2
  Mux3/1 -> Fcn4/1
  Fcn4/1 -> c*/1
  Fcn2/1 -> a*/1
  Fcn3/1 -> b*/1

== system solarPV_grid_04_04/PLL/PLL ==
  vq : Inport
  Constant3 : Constant  Value=2*pi
  Integrator : Integrator
  Mod : Math  Operator=mod  SignedPower=on  SaturateOnIntegerOverflow=on
  PID Controller : slpidlib/PID Controller  Controller=PI  Form=Parallel  TimeDomain=Continuous-time  UseExternalTs=off  SampleTime=-1  IntegratorMethod=Forward Euler  FilterMethod=Forward Euler  ControllerParametersSource=internal  P=10.69499844156994  I=20.78607806516402  D=0  UseFilter=on  N=100  TunerSelectOption=Transfer Function Based (PID Tuner App)  InitialConditionSource=internal  InitialConditionForIntegrator=0  InitialConditionForFilter=0  DifferentiatorICPrevScaledInput=0  ExternalReset=none  TrackingMode=off  Kt=1  LimitOutput=off  SatLimitsSource=internal  UpperSaturationLimit=inf  LowerSaturationLimit=-inf  LinearizeAsGain=on  AntiWindupMode=none  Kb=1  POutMin=[]  POutMax=[]  IOutMin=[]  IOutMax=[]  DOutMin=[]  DOutMax=[]  NOutMin=[]  NOutMax=[]  SumOutMin=[]  SumOutMax=[]  SaturationOutMin=[]  SaturationOutMax=[]  PParamMin=[]  PParamMax=[]  IParamMin=[]  IParamMax=[]  DParamMin=[]  DParamMax=[]  NParamMin=[]  NParamMax=[]  KbParamMin=[]  KbParamMax=[]  KtParamMin=[]  KtParamMax=[]  KbOutMin=[]  KbOutMax=[]  KtOutMin=[]  KtOutMax=[]  IntegratorOutMin=[]  IntegratorOutMax=[]  FilterOutMin=[]  FilterOutMax=[]  SumI1OutMin=[]  SumI1OutMax=[]  SumI2OutMin=[]  SumI2OutMax=[]  SumI3OutMin=[]  SumI3OutMax=[]  SumI4OutMin=[]  SumI4OutMax=[]  SumDOutMin=[]  SumDOutMax=[]  DifferentiatorOutMin=[]  DifferentiatorOutMax=[]  FilterDiffOutCoefMin=[]  FilterDiffOutCoefMax=[]  ReciprocalOutMin=[]  ReciprocalOutMax=[]  SumDenOutMin=[]  SumDenOutMax=[]  SumNumOutMin=[]  SumNumOutMax=[]  DivideOutMin=[]  DivideOutMax=[]  UdiffTsProdOutMin=[]  UdiffTsProdOutMax=[]  NTsProdOutMin=[]  NTsProdOutMax=[]  UintegralTsProdOutMin=[]  UintegralTsProdOutMax=[]  UngainTsProdOutMin=[]  UngainTsProdOutMax=[]  IntegratorContinuousStateAttributes=''  IntegratorStateMustResolveToSignalObject=off  IntegratorRTWStateStorageClass=Auto  FilterContinuousStateAttributes=''  FilterStateMustResolveToSignalObject=off  FilterRTWStateStorageClass=Auto  ParallelPVariant=InternalParameters  IdealPVariant=Disabled  IVariant=InternalParameters  DVariant=Disabled  IntegratorVariant=Continuous  SatVariant=Disabled  AWVariant=Passthrough  PCopyVariant=Disabled  TRVariant=Disabled  FdbkBlocksVariant=Forward  IdealPFdbkVariant=Disabled  SatFdbkVariant=Disabled  DerivativeFilterVariant=Disabled  NVariant=Disabled  NCopyVariant=Disabled_SignalSpec  FilterICVariant=Disabled  IntegratorICVariant=InternalICs  ExternalResetVariant=Disabled  TRSumVariant=Passthrough  SumFdbkVariant=Disabled  SumVariant=Sum_PI  TsampFilterVariant=InternalTs  TsampNgainVariant=Passthrough  TsampIntegralVariant=Passthrough  ExternalSaturationOutDataTypeStr=Inherit: Same as second input
  Scope : Scope  NumInputPorts=2
  Scope1 : Scope
  Sum4 : Sum  Inputs=+-  InputSameDT=on  SampleTime=100e-6
  Sum8 : Sum  Inputs=|++
  Zero1 : Constant  Value=0
  w_ff : Constant  Value=2*3.14*50
  theta : Outport  VectorParamsAs1DForOutWhenUnconnected=off
  w : Outport  Port=2  VectorParamsAs1DForOutWhenUnconnected=off
  wires:
  PID Controller/1 -> Sum8/1
  w_ff/1 -> Sum8/2
  Mod/1 -> theta/1, Scope1/1
  Zero1/1 -> Scope/2, Sum4/2
  Sum4/1 -> PID Controller/1
  vq/1 -> Scope/1, Sum4/1
  Sum8/1 -> Integrator/1, w/1
  Integrator/1 -> Mod/1
  Constant3/1 -> Mod/2

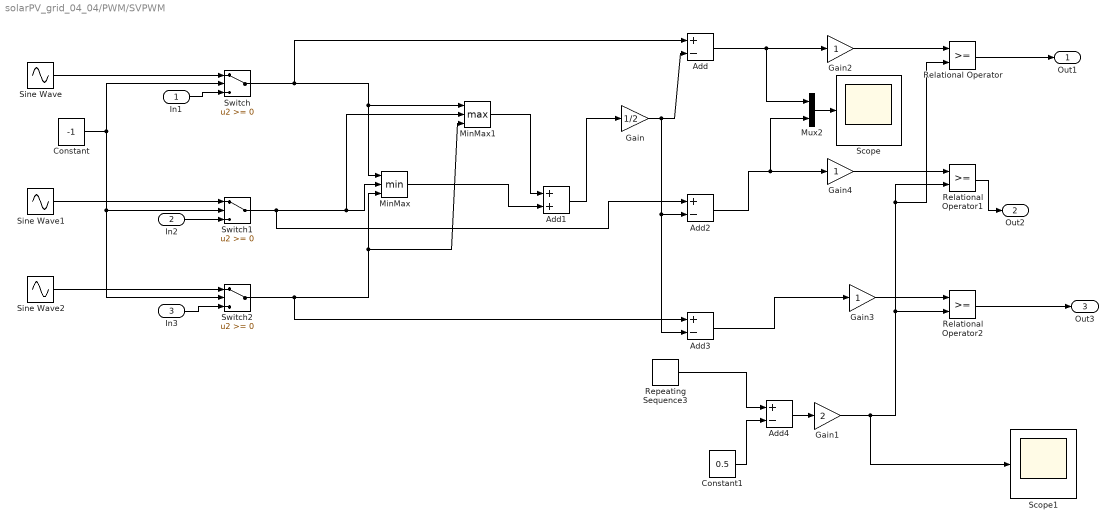
== system solarPV_grid_04_04/PWM/SVPWM ==
  In1 : Inport
  In2 : Inport  Port=2
  In3 : Inport  Port=3
  Add{,2..4} (4 alike) : Sum  Inputs=+-
  Add1 : Sum
  Constant : Constant  Value=-1
  Constant1 : Constant  Value=0.5
  Gain : Gain  Gain=1/2
  Gain1 : Gain  Gain=2
  Gain2 : Gain
  Gain3 : Gain
  Gain4 : Gain
  MinMax : MinMax  Inputs=3
  MinMax1 : MinMax  Function=max  Inputs=3
  Mux2 : Mux  Inputs=2
  Relational Operator : RelationalOperator  OutDataTypeStr=boolean  RndMeth=Nearest
  Relational Operator1 : RelationalOperator  OutDataTypeStr=boolean  RndMeth=Nearest
  Relational Operator2 : RelationalOperator  OutDataTypeStr=boolean  RndMeth=Nearest
  Repeating Sequence3 : simulink/Sources/Repeating Sequence  rep_seq_t=[0 50e-6 100e-6]  rep_seq_y=[0 1 0]
  Scope : Scope
  Scope1 : Scope
  Sine Wave : Sin  Amplitude=5  Frequency=314  SampleTime=0
  Sine Wave1 : Sin  Amplitude=5  Frequency=314  Phase=-2*3.14/3  SampleTime=0
  Sine Wave2 : Sin  Amplitude=5  Frequency=314  Phase=2*3.14/3  SampleTime=0
  Switch : Switch
  Switch1 : Switch
  Switch2 : Switch
  Out1 : Outport
  Out2 : Outport  Port=2
  Out3 : Outport  Port=3
  wires:
  Switch/1 -> Add/1, MinMax/1, MinMax1/1
  Switch1/1 -> MinMax/2, MinMax1/2, Add2/1
  Switch2/1 -> MinMax/3, MinMax1/3, Add3/1
  Gain/1 -> Add2/2, Add3/2, Add/2
  Add/1 -> Gain2/1, Mux2/1
  MinMax1/1 -> Add1/1
  MinMax/1 -> Add1/2
  Add1/1 -> Gain/1
  Add2/1 -> Gain4/1, Mux2/2
  Add3/1 -> Gain3/1
  Constant/1 -> Switch/2, Switch1/2, Switch2/2
  Sine Wave/1 -> Switch/1
  Sine Wave1/1 -> Switch1/1
  Sine Wave2/1 -> Switch2/1
  In1/1 -> Switch/3
  In2/1 -> Switch1/3
  In3/1 -> Switch2/3
  Relational Operator/1 -> Out1/1
  Relational Operator1/1 -> Out2/1
  Relational Operator2/1 -> Out3/1
  Mux2/1 -> Scope/1
  Constant1/1 -> Add4/2
  Repeating Sequence3/1 -> Add4/1
  Add4/1 -> Gain1/1
  Gain1/1 -> Scope1/1, Relational Operator2/2, Relational Operator/2, Relational Operator1/2
  Gain2/1 -> Relational Operator/1
  Gain3/1 -> Relational Operator2/1
  Gain4/1 -> Relational Operator1/1

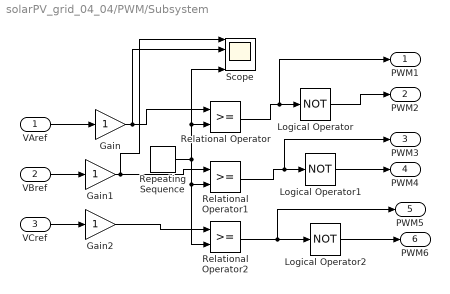
== system solarPV_grid_04_04/PWM/Subsystem ==
  "VAref " : Inport
  VBref : Inport  Port=2
  VCref : Inport  Port=3
  Gain : Gain
  Gain1 : Gain
  Gain2 : Gain
  Logical Operator : Logic  Operator=NOT  AllPortsSameDT=off  OutDataTypeStr=boolean
  Logical Operator1 : Logic  Operator=NOT  AllPortsSameDT=off  OutDataTypeStr=boolean
  Logical Operator2 : Logic  Operator=NOT  AllPortsSameDT=off  OutDataTypeStr=boolean
  Relational Operator : RelationalOperator  OutDataTypeStr=boolean  RndMeth=Simplest
  Relational Operator1 : RelationalOperator  OutDataTypeStr=boolean  RndMeth=Simplest
  Relational Operator2 : RelationalOperator  OutDataTypeStr=boolean  RndMeth=Simplest
  Repeating Sequence : simulink/Sources/Repeating Sequence  rep_seq_t=[0 0.00005 0.0001]  rep_seq_y=[-1 1 -1]
  Scope : Scope  NumInputPorts=4
  PWM1 : Outport  VectorParamsAs1DForOutWhenUnconnected=off
  PWM2 : Outport  Port=2  VectorParamsAs1DForOutWhenUnconnected=off
  PWM3 : Outport  Port=3  VectorParamsAs1DForOutWhenUnconnected=off
  PWM4 : Outport  Port=4  VectorParamsAs1DForOutWhenUnconnected=off
  PWM5 : Outport  Port=5  VectorParamsAs1DForOutWhenUnconnected=off
  PWM6 : Outport  Port=6  VectorParamsAs1DForOutWhenUnconnected=off
  wires:
  Logical Operator/1 -> PWM2/1
  Repeating Sequence/1 -> Relational Operator1/2, Relational Operator2/2, Scope/4, Relational Operator/2
  Relational Operator2/1 -> PWM5/1, Logical Operator2/1
  Relational Operator/1 -> PWM1/1, Logical Operator/1
  Logical Operator1/1 -> PWM4/1
  Relational Operator1/1 -> PWM3/1, Logical Operator1/1
  Logical Operator2/1 -> PWM6/1
  VBref/1 -> Gain1/1
  VCref/1 -> Gain2/1
  "VAref "/1 -> Gain/1
  Gain/1 -> Scope/2, Relational Operator/1
  Gain1/1 -> Scope/1, Relational Operator1/1
  Gain2/1 -> Relational Operator2/1

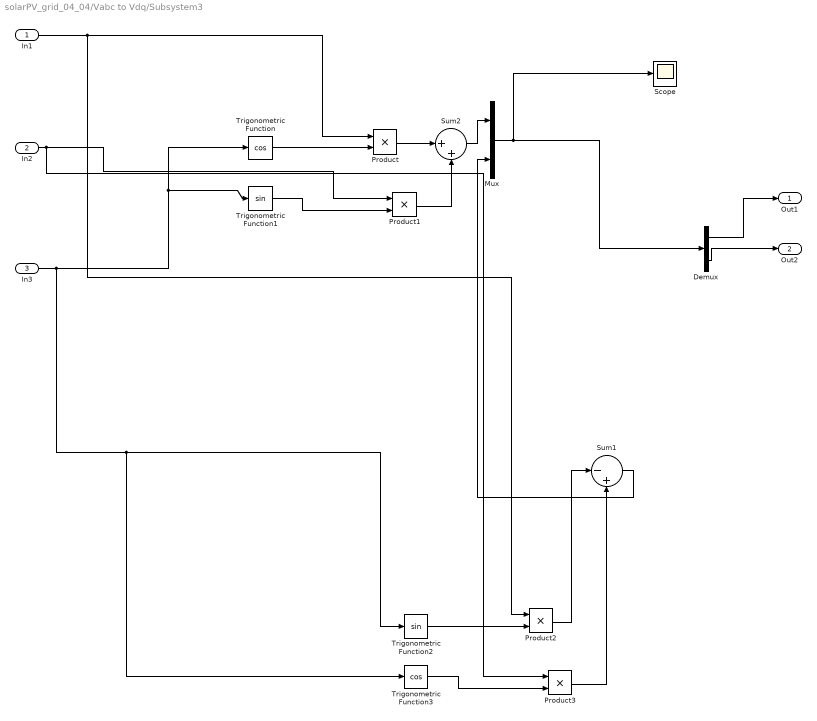
== system solarPV_grid_04_04/Vabc to Vdq/Subsystem3 ==
  In1 : Inport
  In2 : Inport  Port=2
  In3 : Inport  Port=3
  Demux : Demux  Outputs=2
  Mux : Mux  Inputs=2
  Product{,1..3} (4 alike) : Product
  Scope : Scope
  Sum1 : Sum  Inputs=|-+
  Sum2 : Sum  Inputs=|++
  Trigonometric Function : Trigonometry  Operator=cos
  Trigonometric Function1 : Trigonometry
  Trigonometric Function2 : Trigonometry
  Trigonometric Function3 : Trigonometry  Operator=cos
  Out1 : Outport  VectorParamsAs1DForOutWhenUnconnected=off
  Out2 : Outport  Port=2  VectorParamsAs1DForOutWhenUnconnected=off
  wires:
  Demux/1 -> Out1/1
  Demux/2 -> Out2/1
  In3/1 -> Trigonometric Function3/1, Trigonometric Function2/1, Trigonometric Function1/1, Trigonometric Function/1
  Trigonometric Function/1 -> Product/2
  Product/1 -> Sum2/1
  In2/1 -> Product3/1, Product1/1
  Trigonometric Function1/1 -> Product1/2
  Product1/1 -> Sum2/2
  Product3/1 -> Sum1/2
  Product2/1 -> Sum1/1
  Trigonometric Function3/1 -> Product3/2
  Trigonometric Function2/1 -> Product2/2
  In1/1 -> Product2/1, Product/1
  Mux/1 -> Scope/1, Demux/1
  Sum2/1 -> Mux/1
  Sum1/1 -> Mux/2

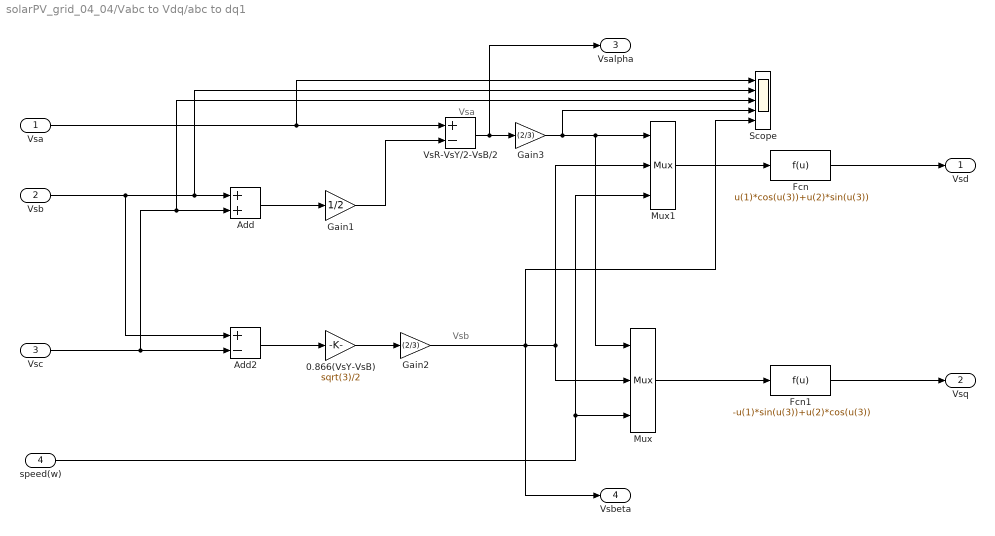
== system solarPV_grid_04_04/Vabc to Vdq/abc to dq1 ==
  note: Vsa
  note: Vsb
  Vsa : Inport
  Vsb : Inport  Port=2
  Vsc : Inport  Port=3
  speed(w) : Inport  Port=4
  0.866(VsY-VsB) : Gain  Gain=sqrt(3)/2
  Add : Sum
  Add2 : Sum  Inputs=+-
  Fcn : Fcn  Expr=u(1)*cos(u(3))+u(2)*sin(u(3))
  Fcn1 : Fcn  Expr=-u(1)*sin(u(3))+u(2)*cos(u(3))
  Gain1 : Gain  Gain=1/2
  Gain2 : Gain  Gain=(2/3)
  Gain3 : Gain  Gain=(2/3)
  Mux : Mux  Inputs=3
  Mux1 : Mux  Inputs=3
  Scope : Scope  NumInputPorts=5
  VsR-VsY/2-VsB/2 : Sum  Inputs=+-
  Vsd : Outport
  Vsq : Outport  Port=2
  Vsalpha : Outport  Port=3
  Vsbeta : Outport  Port=4
  wires:
  speed(w)/1 -> Mux/3, Mux1/3
  VsR-VsY/2-VsB/2/1 -> Gain3/1, Vsalpha/1
  0.866(VsY-VsB)/1 -> Gain2/1
  Fcn1/1 -> Vsq/1
  Fcn/1 -> Vsd/1
  Vsb/1 -> Scope/2, Add/1, Add2/1
  Vsa/1 -> Scope/1, VsR-VsY/2-VsB/2/1
  Vsc/1 -> Add2/2, Scope/3, Add/2
  Add2/1 -> 0.866(VsY-VsB)/1
  Add/1 -> Gain1/1
  Gain1/1 -> VsR-VsY/2-VsB/2/2
  Mux/1 -> Fcn1/1
  Mux1/1 -> Fcn/1
  Gain3/1 -> Scope/4, Mux1/1, Mux/1
  Gain2/1 -> Scope/5, Mux/2, Mux1/2, Vsbeta/1

== matlab function solarPV_grid_04_04/POMPP ==
  data: Vpv input; Vdc_ref output; Ipv input; del input; power output
function [Vdc_ref,power] = fcn(Vpv,Ipv,del)

Vdc_init=700;
Vdc_min=650;
Vdc_max=750;

persistent Vpvold Ppvold vdc_old;

if isempty(Vpvold)

Vpvold=0;
Ppvold=0;
vdc_old=Vdc_init;
end

P=Vpv*Ipv;
dv=Vpv-Vpvold;
dp=P-Ppvold;

if(dp<0)
    t=-dp;
else
    t=dp;
end

if (t >1 && Vpv>650 )
    
    if (dp<0)
        if (dv<0)
            Vdc_ref=vdc_old+del;
        else
            Vdc_ref=vdc_old-del;
            
        end
    else
         if (dv<0)
            Vdc_ref=vdc_old-del;
        else
            Vdc_ref=vdc_old+del;
            
         end
    end
else
    Vdc_ref=vdc_old;
end

if (Vdc_ref>Vdc_max)
    
    Vdc_ref=Vdc_max;
    
elseif (Vdc_ref<Vdc_min)
    
    Vdc_ref=Vdc_min;
end   
Vpvold=Vpv;
Ppvold=P;
vdc_old=Vdc_ref;
power=Ppvold;

== matlab function solarPV_grid_04_04/MATLAB Function ==
  data: Vpv input; Vdc_ref output; Ipv input; del input
function Vdc_ref = fcn(Vpv,Ipv,del)

Vdc_init=4;
Vdc_min=-10;
Vdc_max=0;

persistent Vpvold Ppvold vdc_old;

if isempty(Vpvold)

Vpvold=0;
Ppvold=0;
vdc_old=Vdc_init;
end

P=Vpv*Ipv;
dv=Vpv-Vpvold;
dp=P-Ppvold;

if (dp ~=0 && Vpv>650)
    
    if (dp<0)
        if (dv<0)
            Vdc_ref=vdc_old-del;
        else
            Vdc_ref=vdc_old+del;
            
        end
    else
         if (dv<0)
            Vdc_ref=vdc_old+del;
        else
            Vdc_ref=vdc_old-del;
            
         end
    end
else
    Vdc_ref=vdc_old;
end

if (Vdc_ref>Vdc_max)
    
    Vdc_ref=Vdc_max;
    
elseif (Vdc_ref<Vdc_min)
    
    Vdc_ref=Vdc_min;
end   
Vpvold=Vpv;
Ppvold=P;
vdc_old=Vdc_ref;
